simulink model "WritingRobot"  (R2021a)
settings: Solver=VariableStepAuto  StartTime=0.0  StopTime=30  RelTol=1e-3
model workspace: external: MATLAB File C:\Users\RrPi\Desktop\Robots\WritingRobotV3\WritingRobot_DataFile.m (data not in the file)
values from neighbouring files (symbols this model uses):
  waypoints_Visuals_L = [ ... (first row only)    [WritingRobotV3Code.m]
undefined symbols (not defined in the file or in its folder): smiData, X, Y, Z
libraries: sm_lib x56, nesl_utility x17, robotcorelib x1
(part 2 of 2)

== matlab function WritingRobot/Forward Dynamics ==
  data: d_1 input; tau_1 output; theta_1 input; theta_2 input; tau_2 output; dd_1 input; dtheta_1 input; dtheta_2 input; ddd_1 input; ddtheta_1 input; ddtheta_2 input; tau_3 output
function [tau_1, tau_2, tau_3] = Dynamics(d_1,theta_1,theta_2,dd_1,dtheta_1,dtheta_2,ddd_1, ddtheta_1,ddtheta_2)

m_1=7.49980007;
m_2=8.651076019;
m_3=8.651076019; 

l_1=0.1;
l=0.48; % l=l_2=l_3=0.48

g=9.80665;

% Declare trigonometric functions
theta_1_90=theta_1+pi/2;

c_1=cos(theta_1_90);
c_2=cos(theta_2);
c_12=cos(theta_1_90+theta_2);

s_1=sin(theta_1_90);
s_2=sin(theta_2);
s_12=sin(theta_1_90+theta_2);

% Acceleration-Related Symmetric Matrix
D_11 = m_1+m_2+m_3;

D_12 =-(1/2)*l*m_2*c_2+c_1*l*m_3+(3/2)*l*m_3*c_12;

D_13 =(3/2)*l*m_3*c_12;

D_22=(1/3)*l^2*m_2*s_1^2+(1/3)*l^2*m_2*c_1^2+(1/3)*l^2*m_3*c_12^2+l^2*m_3*s_1^2+...
    l^2*m_3*s_1*c_12+l^2*m_3*s_12^2+l^2*m_3*s_12*c_12+2*l^2*m_3*s_1*s_12+...
    +l^2*m_3*c_1^2+(1/3)*l^2*m_3*c_12^2+l^2*m_3*c_1*c_12;

D_23=(1/3)*l^2*m_3*c_12^2+(1/2)*l^2*m_3*s_1*c_12+l^2*m_3*s_12^2+l^2*m_3*s_12*c_12+...
    l^2*m_3*s_1*s_12+(1/3)*l^2*m_3*c_12^2+(1/2)*l^2*m_3*c_1*c_12;

D_33=(2/3)*l^2*m_3*c_12^2+l^2*m_3*s_12^2+l^2*m_3*c_12*s_12;

% Coriolis and centrifugal terms
h_1 = 0; % no coriolis or centrifugal effect to the prismatic joint
h_2 = -(1/2)*m_2*s_2*l^2*dtheta_2^2-m_2*s_2*l^2*dtheta_1*dtheta_2;
h_3 = (1/2)*m_2*s_2*l^2*dtheta_1^2;

% Gravity terms
c_1 = 0;
c_2 = -(1/2)*m_1*g*l*c_1-(1/2)*m_2*g*l*c_12-m_2*g*l*c_1;
c_3 = -l*g*m_3*c_12;

%Multiplication of matrices
D_matrix=[D_11, D_12, D_13;
          D_12, D_22, D_23;
          D_13, D_23, D_33];
      
q_dd = [ddd_1; ddtheta_1; ddtheta_2];

h_matrix = [h_1; h_2; h_3];

q_d = [dd_1; dtheta_1; dtheta_2];

c_matrix = [c_1; c_2; c_3];

M_matrix = D_matrix * q_dd;

%torques
torques = M_matrix + h_matrix + c_matrix;
tau_1 = torques(1);
tau_2 = torques(2);
tau_3 = torques(3);
end

== matlab function WritingRobot/forwardKinematics ==
  data: x output; d1 input; y output; theta1 input; theta2 input; theta3 input; z output
function [x, y, z] = forward_kinematics(d1, theta1, theta2, theta3)
x = - 0.48*cos(theta1 + theta2 + 1.5707963267948966192313216916398) - 0.206*cos(theta1 + theta2 + theta3 + 1.5707963267948966192313216916398) - 0.48*cos(theta1 + 1.5707963267948966192313216916398);
y = d1 + 0.2915;
z = 0.48*sin(theta1 + theta2 + 1.5707963267948966192313216916398) + 0.206*sin(theta1 + theta2 + theta3 + 1.5707963267948966192313216916398) + 0.48*cos(theta1 - 1.4420985131352750410631430775095e-33) + 0.1775;
end

== matlab function WritingRobot/inverseKinematics ==
  data: x input; d1 output; y input; z input; theta1 output; theta2 output; theta3 output
function [d1,theta1,theta2,theta3] = inverse_kinematics(x,y,z)
d1=y-0.2915;
theta_total = pi/2;
x_1 = (x)-0.206*sin(theta_total);
z_1 = (z-0.1775)-0.206*cos(theta_total);
theta2 = acos(((x_1^2+z_1^2)-(2*0.48^2))/(2*0.48^2));
theta1 = atan(x_1/z_1) - atan((0.48*sin(theta2))/(0.48+(0.48*cos(theta2))));
theta3 = theta_total - (theta1 + theta2);
end
